simulink library "gavrt_library"  (Simulink 6.2)
libraries: xbsIndex_r3 x217, xps_library x15, casper_library x12, gavrt_library x8
(part 1 of 3)
settings Model: LastModifiedBy=Glenn

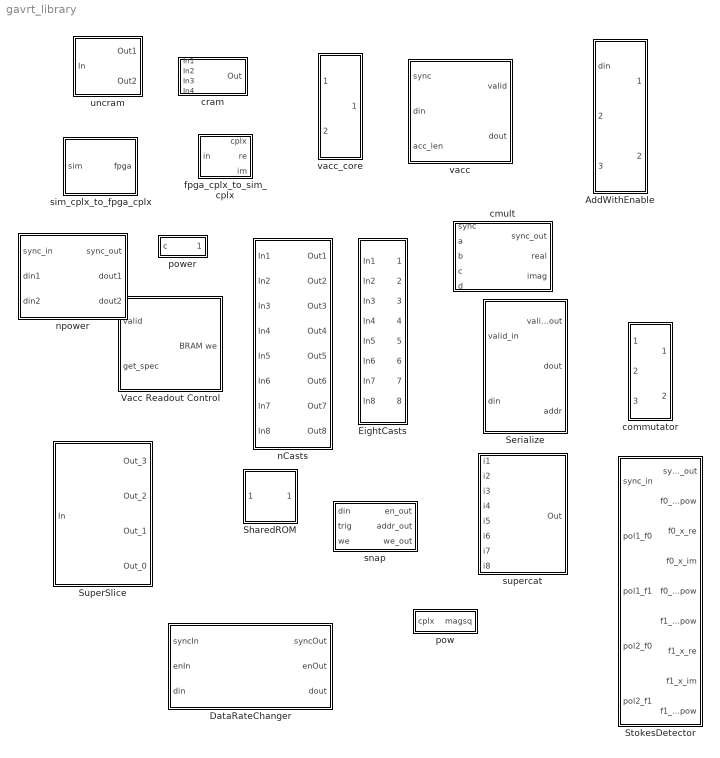
== system gavrt_library ==
  AddWithEnable : Subsystem  mask{acc_width=18, bin_pt=17, add_latency=1}
      mask prompts: acc_width "Output bit width"; bin_pt "Binary Point"; add_latency "Add Latency"
      mask help:
      | Adder with enable.
      | Used by the Addressable accumulator addracc.
      | toram = din + accen * fromram  (with latency add_latency)
      | rdout is for debugging
  DataRateChanger : Subsystem  mask(dataratechanger){input_length=3, ninputs=1, out_rate=1, in_bit_width=8, in_bin_pt=0, arith_type=0}
      mask prompts: input_length "Input Length (2^?)"; ninputs "Number of Simultaneous Inputs (2^?)"; out_rate "Output Rate (2^-?)"; in_bit_width "Input Bit Width"; in_bin_pt "Input Binary Point"; arith_type "Arithmetic Type (0=Unsigned, 1=Signed)"
      mask help:
      | Stores input data into a FIFO and then outputs the data at the specified data rate, cycling through inputs.
      | Thus if the input data looks like:
      | x0 x1 x2 x3 ...
      | y0 y1 y2 y3 ...
      | And the output rate is 2^-1, the output will look like this:
      | x0 x0 y0 y0 x1 x1 y1 y1 x2 x2 y2 y2...
      | enIn (enable In) should be high for 2^Input length clocks while the input data is valid.
      | *Currently enIn must be high in one burst of 2^Input length*
      | din should be all simultaneous inputs "crammed" together
      | enOut will be high for 2^(Input Length + Output Rate + Number of Simultaneous Inputs)
      | Arithmetic type and binary precision is only used for "uncramming" the input data
      mask init:
      | dataratechanger_init(gcb, 'input_length', input_length,...
      |     'ninputs', ninputs, ...
      |     'out_rate', out_rate,...
      |     'in_bit_width', in_bit_width,...
      |     'in_bin_pt', in_bin_pt,...
      |     'arith_type',arith_type);
  EightCasts : Subsystem  mask{nbits=0, bin_pt=0}
      mask prompts: nbits "Number of bits"; bin_pt "Binary Point"
      mask help: Eight casts to quickly connect ADC to FFT
  Serialize : Subsystem  mask(serialize){ninputs=8, in_width=8, depth=32, mux_latency=2}
      mask prompts: ninputs "Number of simultaneous inputs"; in_width "Input data bit width"; mux_latency "Mux Latency"
      mask help:
      | Takes concatenated parallel inputs and presents them one by one on dout. Designed to work with the Specacc block directly. valid_in should be high for 'depth' clocks while the data is present on din. After a short delay from when valid_in returns low, valid_out will go high and the first data will be present on dout and addr will be 0. addr increments for each subsequent output data.  dout(0) is the MSB of the first din word.
      | 'depth' must be a power of two and is the length of the input vectors. The output vector will be ninputs*depth long
      | This block can be directly connected to a Shared BRAM (provided dout is <= 32 bits).
      mask init:
      | serialize_init(gcb, ...
      |     'ninputs', ninputs, ...
      |     'in_width', in_width, ...
      |     'depth', depth, ...
      |     'mux_latency', mux_latency);
  SharedROM : Subsystem  mask(sharedrom){outwidth=327, depth=8192}
      mask prompts: outwidth "Output Bit Width"
      mask init:
      | sharedrom_init(gcb,...
      |     'outwidth', outwidth,...
      |     'depth', depth);
  StokesDetector : Subsystem  mask(stokes){bit_width=18, add_latency=2, mult_latency=3}
      mask prompts: bit_width "Bit Width"; add_latency "Add Latency"; mult_latency "Mult Latency"
      mask help: Compute cross products necessary for full stokes parameters
  SuperSlice : Subsystem  mask(superslice){slices=-1*ones(1,4)}
      mask prompts: slices "Slice pattern"
      mask help:
      | Slices the input word into consecutive outputs of arbitrary width.
      | Slice pattern should be a vector with each entry representing the width of that particular slice. The first entry is the MSB slice and the last is the LSB slice.
      | If a slice is given width -1, that slice will have a boolean output.
      | Ex: -1*ones(1,32)  -- Slice a 32 bit word into seperate boolean flags
      | [16, 8, -1*ones(1,8)] -- Slice a 32 bit word into the MSW, a byte, and the least significant 8 bits
      mask init:
      | superslice_init(gcb, 'slices', slices);
  Vacc Readout Control : Subsystem
      mask Description:
      | Designed for easily reading out vacc block with the PowerPC. Connect valid to the valid out of the vacc or serializer. Connect BRAM we to the we port of the Shared BRAM and make this bit available in a software register. Connect get_spec to a bit from a software register.
      | To read out an accumulation,
      | set get_spec high
      | wait for BRAM we to go low
      | read valid accumulation from Shared BRAM
      | set get_spec low
  cmult : Subsystem  mask(cmult_em){mult_latency=4, add_latency=3}
      mask prompts: mult_latency "Mult Latency"; add_latency "Add Latency"
      mask help: Perform a complex multiplication (a+bi)(c-di)=(ac-bd)+(ad+bc)i. Implements the logic in embedded multipliers.
  commutator : Subsystem  mask(commutator){ninputs=8, in_width=32, mux_latency=2}
      mask prompts: ninputs "Number of inputs"; in_width "Input width"; mux_latency "Mux Latency"
      mask help:
      | Used by the Serialize block.
      | din is concatenated parallel inputs. dout commutates through din from MSB to LSB.
      mask init:
      | commutator_init(gcb, ...
      |     'ninputs', ninputs, ...
      |     'in_width', in_width, ...
      |     'mux_latency', mux_latency);
  cram : Subsystem  mask(cram){num_slice=4}
      mask prompts: num_slice "Number of slices"
      mask help: Concatenates inputs together after forcing binary point to zero.
      mask init:
      | cram_init(gcb, ...
      |     'num_slice', num_slice);
  fpga_cplx_to_sim_cplx : Subsystem  mask{width=18}
      mask prompts: width "Data Width"
      mask help: Converts a Casper complex to a Simulink complex
      mask init:
      | set_param(gcb, 'AttributesFormatString', sprintf('%d_%d bit',width,width-1));
      settings: AttributesFormatString=18_17 bit
  nCasts : Subsystem  mask(ncasts){ncasts=8, arith_type=0, nbits=8, bin_pt=3}
      mask prompts: ncasts "Number of Casts"; arith_type "Arithmetic Type (0=Unsigned, 1=Signed, 2=Boolean)"; nbits "Output Bit Width"; bin_pt "Binary Point"
      mask init:
      | ncasts_init(gcb, ...
      |     'ncasts', ncasts, ...
      |     'arith_type', arith_type, ...
      |     'nbits', nbits, ...
      |     'bin_pt', bin_pt);
  npower : Subsystem  mask(npower){n_inputs=2, in_width=18, add_latency=2, mult_latency=3}
      mask prompts: n_inputs "Number of inputs"; in_width "Input Bit Width"; add_latency "Add Latency"; mult_latency "Mult Latency"
      mask init:
      | npower_init(gcb, ...
      |     'n_inputs', n_inputs, ...
      |     'in_width', in_width, ...
      |     'add_latency', add_latency, ...
      |     'mult_latency', mult_latency)
      settings: AttributesFormatString=latency=5
  pow : Subsystem  mask{bit_width=18, add_latency=2, mult_latency=3}
      mask prompts: bit_width "Bit Width"; add_latency "Add Latency"; mult_latency "Mult Latency"
  power : Subsystem  mask{BitWidth=18, add_latency=2, mult_latency=3}
      mask prompts: BitWidth "Bit Width"; add_latency "Add Latency"; mult_latency "Mult Latency"
  sim_cplx_to_fpga_cplx : Subsystem  mask{width=18}
      mask prompts: width "Data Width"
      mask help:
      | Converts a Simulink complex to fixed point and concatenates it to a Casper complex.
      | Output is two Fix_width_(width-1) numbers concatenated.
      mask init:
      | set_param(gcb, 'AttributesFormatString', sprintf('%d_%d bit',width,width-1));
      settings: AttributesFormatString=18_17 bit
  snap : Subsystem  mask(snap64){nsamples=13, latency=4}
      mask prompts: nsamples "No. of samples(2^?)"; latency "Register Latency"
      mask help:
      | The <i>snap</i> block provides a packaged solution to capturing data from
      | the FPGA fabric and making it accessible from the CPU.  The block comes in
      | 2 flavors: <i>snap</i> (which captures to a 32 bit wide Shared BRAM), and
      | <i>snap64</i> (which captures to 2x32 bit wide Shared BRAMs to effect a
      | 64 bit capture).
      | en_out provides access to the ctrl[en] bit
      | addr_out and we_out can be used to control additional BRAMs to allow for wider captures than 64 bits.
      | Register latency specifies how many levels of registers to use between the control logic and the software registers and Shared BRAMs. Adding latency can help timing when compiling at 250 MHz
      mask Help: eval('xlWeb([getenv(''MLIB_ROOT''), ''\casper_library\doc\snap_usage.html''])')
  supercat : Subsystem  mask(supercat){n=8}
      mask prompts: n "Number of Inputs"
      mask init:
      | supercat_init(gcb, 'n', n);
  uncram : Subsystem  mask(uncram){num_slice=2, slice_width=18, bin_pt=17, arith_type=1}
      mask prompts: num_slice "Number of slices"; slice_width "Slice Width"; bin_pt "Output Binary Point"; arith_type "Output Arithmetic Type (0=Unsigned, 1=Signed)"
      mask help: Takes a concatenated input and slices it up into even pieces and reinterprets them as signed fixed point numbers with a given binary point.
      mask init:
      | uncram_init(gcb, ...
      |     'num_slice', num_slice, ...
      |     'slice_width', slice_width, ...
      |     'bin_pt', bin_pt, ...
      |     'arith_type', arith_type);
      settings: AttributesFormatString=Fix_18_17
  vacc : Subsystem  mask(vacc){veclen=8, ninputs=4, max_accum=16, arith_type=0, in_bit_width=32, in_bin_pt=31, out_bit_width=48, out_bin_pt=31, register_din=0, add_latency=2, bram_latency=2, mux_latency=1}
      mask prompts: veclen "Vector Length (2^?)"; ninputs "Number of Simultaneous Vectors"; max_accum "Maximum # Accumulations (2^?)"; arith_type "Arithmetic Type (0=Unsigned, 1=Signed)"; in_bit_width "Input Bit Width"; in_bin_pt "Input Binary Point"; out_bit_width "Output Bit Width"; out_bin_pt "Output Binary Point"; register_din "Register Input Data  (1 = Enable Register Retiming on input delay)"; add_latency "Add Latency"; bram_latency "BRAM Latency"; mux_latency "Mux Latency"
      mask help:
      | Sync is expected the clock before the first data to be accumulated.
      | Use the Cram block to feed din for multiple simultaneous inputs.
      | acc_len is the number of vectors to sum.
      | valid is high while a valid accumulation is being clocked out on dout.
      | If only one sync pulse is provided, valid accumulations will repeatedly appear on dout as they become available.
      | Undesired behavior may occur if acc_len is changed without a new sync pulse.
      | Note: The output is an unsigned concatenation of the output streams. Thus, even with only one stream, the output must be recast before using.
      | Register Input Data controls the "Enable Register Retiming" parameter of the delays on 'din'.
      mask init:
      | vacc_init(gcb, ...
      |     'veclen', veclen, ...
      |     'ninputs', ninputs, ...
      |     'max_accum', max_accum, ...
      |     'arith_type', arith_type, ...
      |     'in_bit_width', in_bit_width, ...
      |     'in_bin_pt', in_bin_pt, ...
      |     'out_bit_width', out_bit_width, ...
      |     'out_bin_pt', out_bin_pt, ...
      |     'register_din', register_din, ...
      |     'add_latency', add_latency, ...
      |     'bram_latency', bram_latency, ...
      |     'mux_latency', mux_latency);
      settings: AttributesFormatString=|
      | vector length=256, inputs=4
      | max accumulations=2^16
  vacc_core : Subsystem  mask(vacc_core){veclen=16, arith_type=0, out_bit_width=14, out_bin_pt=0, add_latency=2, bram_latency=2, mux_latency=1}
      mask prompts: veclen "Vector Length"; arith_type "Arithmetic Type (0=Unsigned, 1=Signed)"; out_bit_width "Output Bit Width"; out_bin_pt "Output Binary Point"; add_latency "Add Latency"; bram_latency "BRAM Latency"; mux_latency "Mux Latency"
      mask help:
      | Currently only Signed arithmetic supported
      | acc_en = 0 --> Load a vector (start a new accumulation)
      | acc_en = 1 --> Accumulate
      mask init:
      | vacc_core_init(gcb, ...
      |     'veclen', veclen, ...
      |     'arith_type', arith_type, ...
      |     'out_bit_width', out_bit_width, ...
      |     'out_bin_pt', out_bin_pt, ...
      |     'add_latency', add_latency, ...
      |     'bram_latency', bram_latency, ...
      |     'mux_latency', mux_latency);

== system gavrt_library/AddWithEnable ==
  din : Inport  Port=1  LatchInput=off
  accen : Inport  Port=2  LatchInput=off
  fromram : Inport  Port=3  LatchInput=off
  AddSub : xbsIndex_r3/AddSub  mode=Addition  precision=Full  arith_type=Unsigned  n_bits=8  bin_pt=2  quantization=Truncate  overflow=Wrap  latency=add_latency  explicit_period=off  period=1  use_carryin=off  use_carryout=off  en=off  dbl_ovrd=off  show_param=on  use_core=on  pipeline=on  use_rpm=on  gen_core=off
      settings: xl_area=[0, 0, 0, 0, 0, 0, 0]
  Constant1 : xbsIndex_r3/Constant  const=0  equ=P=C  arith_type="Signed  (2's comp)"  n_bits=acc_width  bin_pt=bin_pt  opselect=C  inp2=PCIN>>17  opr=+  inp1=P  carry=CIN  iostate=0  explicit_period=on  period=1  dbl_ovrd=off
  Convert2 : xbsIndex_r3/Convert  arith_type="Signed  (2's comp)"  n_bits=acc_width  bin_pt=bin_pt  quantization=Truncate  overflow=Wrap  latency=0  explicit_period=off  period=1  dbl_ovrd=off  show_param=off  inserted_by_tool=off  pipeline=off
      settings: xl_area=[0, 0, 0, 0, 0, 0, 0]
  Mux : xbsIndex_r3/Mux  inputs=2  precision=Full  arith_type="Signed  (2's comp)"  n_bits=8  bin_pt=2  quantization=Truncate  overflow=Wrap  latency=0  explicit_period=off  period=1  en=off  dbl_ovrd=off  show_param=off  mux_type=off  use_rpm=off  gen_core=off
      settings: xl_area=[0, 0, 0, 0, 0, 0, 0]
  Reinterpret : xbsIndex_r3/Reinterpret  force_arith_type=on  arith_type="Signed  (2's comp)"  force_bin_pt=on  bin_pt=bin_pt  force_valid=on
  Reinterpret1 : xbsIndex_r3/Reinterpret  force_arith_type=on  arith_type=Unsigned  force_bin_pt=on  bin_pt=0  force_valid=on
  toram : Outport
  rdout : Outport  Port=2
  wires:
  Constant1/1 -> Mux/2
  Reinterpret/1 -> Mux/3, rdout/1
  Mux/1 -> AddSub/2
  AddSub/1 -> Convert2/1
  Convert2/1 -> Reinterpret1/1
  din/1 -> AddSub/1
  accen/1 -> Mux/1
  Reinterpret1/1 -> toram/1
  fromram/1 -> Reinterpret/1

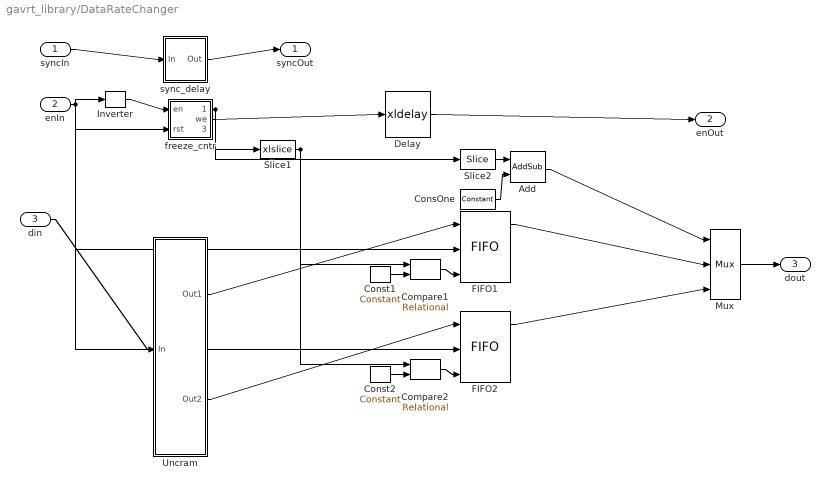
== system gavrt_library/DataRateChanger ==
  syncIn : Inport  Port=1  LatchInput=off
  enIn : Inport  Port=2  LatchInput=off
  din : Inport  Port=3  LatchInput=off
  Add : xbsIndex_r3/AddSub  mode=Addition  precision=User Defined  arith_type=Unsigned  n_bits=1  bin_pt=0  quantization=Truncate  overflow=Wrap  latency=0  explicit_period=off  period=1  use_carryin=off  use_carryout=off  en=off  dbl_ovrd=off  show_param=off  use_core=on  pipeline=off  use_rpm=on  gen_core=off
      settings: xl_area=[0, 0, 0, 0, 0, 0, 0]
  Compare1 : xbsIndex_r3/Relational  mode=a=b  latency=0  explicit_period=off  period=1  en=off  dbl_ovrd=off  show_param=off
      settings: xl_area=[0, 0, 0, 0, 0, 0, 0]
  Compare2 : xbsIndex_r3/Relational  mode=a=b  latency=0  explicit_period=off  period=1  en=off  dbl_ovrd=off  show_param=off
      settings: xl_area=[0, 0, 0, 0, 0, 0, 0]
  ConsOne : xbsIndex_r3/Constant  const=1  equ=P=C  arith_type=Unsigned  n_bits=1  bin_pt=0  opselect=C  inp2=PCIN>>17  opr=+  inp1=P  carry=CIN  iostate=0  explicit_period=off  period=1  dbl_ovrd=off
  Const1 : xbsIndex_r3/Constant  const=1  equ=P=C  arith_type=Unsigned  n_bits=2  bin_pt=0  opselect=C  inp2=PCIN>>17  opr=+  inp1=P  carry=CIN  iostate=0  explicit_period=off  period=1  dbl_ovrd=off
  Const2 : xbsIndex_r3/Constant  const=3  equ=P=C  arith_type=Unsigned  n_bits=2  bin_pt=0  opselect=C  inp2=PCIN>>17  opr=+  inp1=P  carry=CIN  iostate=0  explicit_period=off  period=1  dbl_ovrd=off
  Delay : S-Function  AncestorBlock=xbsIndex_r3/Delay  FunctionName=xldelay  Parameters=sfcn_mwsv__  mask(Xilinx Delay Block){latency=3, reg_retiming=off, explicit_period=off, period=1, en=off, accept_only_valid=off, init_zero=on, dbl_ovrd=off, show_param=off, xl_area=[0, 0, 0, 0, 0, 0, 0], xl_use_area=off}
      mask prompts: reg_retiming "Enable Register Retiming"; explicit_period "Use Explicit Sample Period"; period "Sample Period  (use -1 to inherit first known input period)"; en "Provide Enable Port"; accept_only_valid "Shift In Only Valid Data"; init_zero "Initialize with Zeros (otherwise Invalid)"; dbl_ovrd "Override with Doubles"; show_param "---------------------- Show Implementation Parameters -----------------------------------------------------------------------------------"; xl_area "FPGA Area [Slices, FFs, BRAMs, LUTs, IOBs, Emb. Mults, TBUFs]"; xl_use_area "Use Area Above For Estimation"
      mask help:
      | Delay line having  configurable length.
      |
      | Hardware notes: A delay line is a chain, each link of which is an SRL16 followed by a flip-flop. If register retiming is enabled, the delay line is a chain of flip-flops.
      mask init:
      | rst = 0;
      | [enPortNum,enPortStr,rstPortNum,rstPortStr] = xlport_en_rst(en,rst,2);
      | str = sprintf('-%d',latency);
      | [designRoot, family, part, speed, package, simulinkPeriod, sysclkPeriod, dbl_ovrd, trimVbit] = xlSysgenSettings(gcb,1,1);
      | [bg,fg] = xlcmap('XBlock',dbl_ovrd);
      | iPos = get_param(gcb,'Position');
      | iWidth=iPos(3)-iPos(1); iHeight=iPos(4)-iPos(2);
      | iCx=iWidth/2;
      | iCy=iHeight/2;
      | [logoX, logoY] = xlogo(iPos);
      | 
      | 
      | % one time added for param list
      | dblOvrd = dbl_ovrd;
      | vOnly = accept_only_valid;
      | initZero = init_zero;
      | precision0 = 1;
      | z0 = [0 0 1 1 1];
      | explicitClk = explicit_period;
      | 
      | hasRST = rst;
      | hasEN = en;
      | % just pass everything to s-function
      | sfcn_mwsv__ = get_param(gcb, 'MaskWSVariables');
      mask Help: eval('xlWeb(xlhtmldoclink(''Delay''))');
      mask CallbackString: ||xlMagicCallback||||||xlShowIPCallback||
      mask Display:
      | patch([0 iWidth iWidth 0],[0 0 iHeight iHeight] , bg);
      | patch(logoX,logoY , fg);
      | text(iCx-6,iCy,'z');
      | text(iCx,iCy+4,str);
      | port_label('input',enPortNum,enPortStr);
      | ;plot([0 0 iWidth iWidth 0], [0 iHeight iHeight 0 0]);
  FIFO1 : xbsIndex_r3/FIFO  depth=16  percent_nbits=1  store_only_valid=on  init_zero=on  explicit_period=off  period=1  rst=off  en=off  use_almost_empty=off  almost_empty_offset=6  use_almost_full=off  almost_full_offset=6  dbl_ovrd=off  show_param=off  mem_type=Block RAM  gen_core=off
      settings: xl_area=[0, 0, 0, 0, 0, 0, 0]
  FIFO2 : xbsIndex_r3/FIFO  depth=16  percent_nbits=1  store_only_valid=on  init_zero=on  explicit_period=off  period=1  rst=off  en=off  use_almost_empty=off  almost_empty_offset=6  use_almost_full=off  almost_full_offset=6  dbl_ovrd=off  show_param=off  mem_type=Block RAM  gen_core=off
      settings: xl_area=[0, 0, 0, 0, 0, 0, 0]
  Inverter : xbsIndex_r3/Inverter  latency=0  explicit_period=off  period=1  en=off  dbl_ovrd=off  show_param=off
      settings: xl_area=[0, 0, 0, 0, 0, 0, 0]
  Mux : xbsIndex_r3/Mux  inputs=2  precision=Full  arith_type="Signed  (2's comp)"  n_bits=8  bin_pt=2  quantization=Truncate  overflow=Wrap  latency=1  explicit_period=off  period=1  en=off  dbl_ovrd=off  show_param=off  mux_type=off  use_rpm=off  gen_core=off
      settings: xl_area=[0, 0, 0, 0, 0, 0, 0]
  Slice1 : S-Function  AncestorBlock=xbsIndex_r3/Slice  FunctionName=xlslice  Parameters=sfcn_mwsv__  mask(Xilinx Slice Block){mode=Lower Bit Location + Width, nbits=2, bit1=-3, base1=MSB of Input, bit0=0, base0=LSB of Input, boolean_output=off, explicit_period=off, period=1, dbl_ovrd=off}
      mask prompts: mode "Specify Range As"; nbits "Width of Slice (number of bits)"; bit1 "Offset of Top Bit"; base1 "Relative To"; bit0 "Offset of Bottom Bit"; base0 "Relative To"; boolean_output "Boolean Output"; explicit_period "Use Explicit Sample Period"; period "Sample Period"; dbl_ovrd "Override with Doubles"
      mask help:
      | Bit slice extractor.  Extracts a given range of bits from each input sample and presents it at the output.  The output type is ordinarily unsigned with binary point at zero, but can be Boolean when the slice is one bit wide.
      |
      | Hardware notes: In hardware this block costs nothing.
      mask init:
      | [designRoot, family, part, speed, package, simulinkPeriod, sysclkPeriod, dbl_ovrd, trimVbit] = xlSysgenSettings(gcb,1,1);
      | dbl_ovrdStr = '';
      | [bg,fg]=xlcmap('XBlock',dbl_ovrd);
      | iPos = get_param(gcb,'Position');
      | iWidth=iPos(3)-iPos(1); iHeight=iPos(4)-iPos(2);
      | iCx=iWidth/2;
      | iCy=iHeight/2;
      | [logoX, logoY] = xlogo(iPos);
      | 
      | 
      | % one time added for param list
      | bo = boolean_output;
      | dblOvrd = dbl_ovrd;
      | precision0 = 1;
      | z0 = [nbits 0 1 1 1];
      | explicitClk = explicit_period;
      | 
      | 
      | % just pass everything to s-function
      | sfcn_mwsv__ = get_param(gcb, 'MaskWSVariables');
      mask Help: eval('xlWeb(xlhtmldoclink(''Slice''))');
      mask StyleString: popup(Two Bit Locations|Upper Bit Location + Width|Lower Bit Location + Width),edit,edit,popup(LSB of Input|Binary Point of Input|MSB of Input),edit,popup(LSB of Input|Binary Point of Input|MSB of Input),checkbox,checkbox,edit,checkbox
      mask CallbackString: xlslice_callback|||||||xlMagicCallback||
      mask Display:
      | patch([0 iWidth iWidth 0],[0 0 iHeight iHeight] , bg);
      | patch(logoX,logoY , fg);
      | port_label('output',1,'[a:b]');
      | 
      | ;plot([0 0 iWidth iWidth 0], [0 iHeight iHeight 0 0]);
  Slice2 : xbsIndex_r3/Slice  mode=Lower Bit Location + Width  nbits=1  bit1=0  base1=MSB of Input  bit0=1  base0=LSB of Input  boolean_output=off  explicit_period=off  period=1  dbl_ovrd=off
  Uncram : Subsystem  AncestorBlock=gavrt_library/uncram  mask(uncram){num_slice=2, slice_width=8, bin_pt=0, arith_type=0}
      mask prompts: num_slice "Number of slices"; slice_width "Slice Width"; bin_pt "Output Binary Point"; arith_type "Output Arithmetic Type (0=Unsigned, 1=Signed)"
      mask help: Takes a concatenated input and slices it up into even pieces and reinterprets them as signed fixed point numbers with a given binary point.
      mask init:
      | uncram_init(gcb, ...
      |     'num_slice', num_slice, ...
      |     'slice_width', slice_width, ...
      |     'bin_pt', bin_pt, ...
      |     'arith_type', arith_type);
      settings: AttributesFormatString=UFix_8_0
  freeze_cntr : Subsystem  AncestorBlock=casper_library/Misc/freeze_cntr  mask(freeze_cntr){CounterBits=5}
      mask prompts: CounterBits "Counter Length (2^?)"
      mask help:
      | A freeze counter is an enabled counter which holds its final value (regardless of enables)
      | until it is reset.
      mask Help: eval('xlWeb([getenv(''MLIB_ROOT''), ''\casper_library\doc\freeze_cntr_usage.html''])')
  sync_delay : Subsystem  AncestorBlock=casper_library/Delays/sync_delay  mask(sync_delay){DelayLen=11}
      mask prompts: DelayLen "Delay Length:"
      mask help: Delay an infrequent boolean pulse by the specified number of clocks.
      mask init:
      | BitWidth = max(2, ceil(log2(DelayLen+1)));
      | UseCounter = 1;
      | if DelayLen == 0,
      | 	UseCounter = 0;
      | end
      mask Help: eval('xlWeb([getenv(''MLIB_ROOT''), ''\casper_library\doc\sync_delay_usage.html''])')
      mask Display: fprintf('Z^-%d', DelayLen)
  syncOut : Outport
  enOut : Outport  Port=2
  dout : Outport  Port=3
  wires:
  FIFO2/1 -> Mux/3
  Uncram/2(Out2) -> FIFO2/1
  Compare2/1 -> FIFO2/3
  Const2/1 -> Compare2/2
  Slice1/1 -> Compare2/1, Compare1/1
  FIFO1/1 -> Mux/2
  Uncram/1(Out1) -> FIFO1/1
  Compare1/1 -> FIFO1/3
  Const1/1 -> Compare1/2
  Add/1 -> Mux/1
  ConsOne/1 -> Add/2
  Slice2/1 -> Add/1
  Mux/1 -> dout/1
  din/1 -> Uncram/1(In)
  freeze_cntr/1(addr) -> Slice2/1, Slice1/1
  Delay/1 -> enOut/1
  freeze_cntr/2(we) -> Delay/1
  Inverter/1 -> freeze_cntr/1(en)
  enIn/1 -> FIFO2/2, FIFO1/2, freeze_cntr/2(rst), Inverter/1
  sync_delay/1(Out) -> syncOut/1
  syncIn/1 -> sync_delay/1(In)

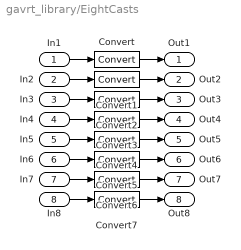
== system gavrt_library/EightCasts ==
  In1 : Inport  Port=1  LatchInput=off
  In2 : Inport  Port=2  LatchInput=off
  In3 : Inport  Port=3  LatchInput=off
  In4 : Inport  Port=4  LatchInput=off
  In5 : Inport  Port=5  LatchInput=off
  In6 : Inport  Port=6  LatchInput=off
  In7 : Inport  Port=7  LatchInput=off
  In8 : Inport  Port=8  LatchInput=off
  Convert{,1..7} (8 alike) : xbsIndex_r3/Convert  arith_type="Signed  (2's comp)"  n_bits=nbits  bin_pt=bin_pt  quantization=Truncate  overflow=Wrap  latency=0  explicit_period=off  period=1  dbl_ovrd=off  show_param=off  inserted_by_tool=off  pipeline=off
      settings: xl_area=[0, 0, 0, 0, 0, 0, 0]
  Out1 : Outport
  Out2 : Outport  Port=2
  Out3 : Outport  Port=3
  Out4 : Outport  Port=4
  Out5 : Outport  Port=5
  Out6 : Outport  Port=6
  Out7 : Outport  Port=7
  Out8 : Outport  Port=8
  wires:
  Convert7/1 -> Out8/1
  In8/1 -> Convert7/1
  Convert6/1 -> Out7/1
  In7/1 -> Convert6/1
  Convert5/1 -> Out6/1
  In6/1 -> Convert5/1
  Convert4/1 -> Out5/1
  In5/1 -> Convert4/1
  Convert3/1 -> Out4/1
  In4/1 -> Convert3/1
  Convert2/1 -> Out3/1
  In3/1 -> Convert2/1
  Convert1/1 -> Out2/1
  In2/1 -> Convert1/1
  Convert/1 -> Out1/1
  In1/1 -> Convert/1

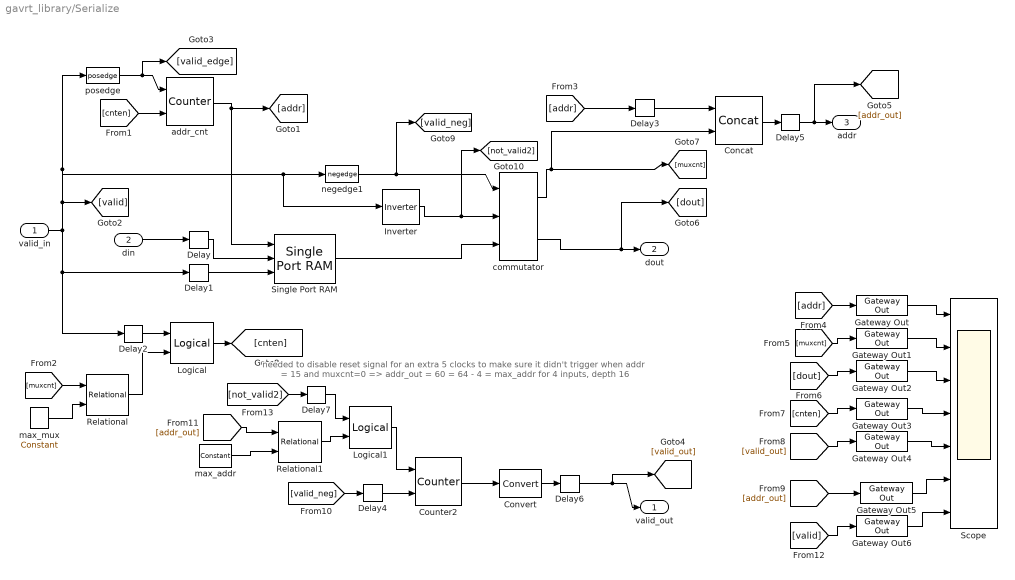
== system gavrt_library/Serialize ==
  note: needed to disable reset signal for
      | an extra 5 clocks to make sure it didn't
      | trigger when addr = 15 and muxcnt=0 =>
      | addr_out = 60 = 64 - 4 = max_addr for
      | 4 inputs, depth 16
  valid_in : Inport  Port=1  LatchInput=off
  din : Inport  Port=2  LatchInput=off
  Concat : xbsIndex_r3/Concat  num_inputs=2  explicit_period=off  period=1  dbl_ovrd=off
  Convert : xbsIndex_r3/Convert  arith_type=Boolean  n_bits=8  bin_pt=6  quantization=Truncate  overflow=Wrap  latency=0  explicit_period=off  period=1  dbl_ovrd=off  show_param=off  inserted_by_tool=off  pipeline=off
      settings: xl_area=[0, 0, 0, 0, 0, 0, 0]
  Counter2 : xbsIndex_r3/Counter  cnt_type=Free Running  n_bits=1  bin_pt=0  arith_type=Unsigned  start_count=0  cnt_to=Inf  cnt_by_val=1  operation=Up  explicit_period=off  period=1  load_pin=off  rst=on  en=on  dbl_ovrd=off  show_param=off  use_rpm=on  gen_core=off
      settings: xl_area=[0, 0, 0, 0, 0, 0, 0]
  Delay{,1..4} (5 alike) : xbsIndex_r3/Delay  latency=1  reg_retiming=off  explicit_period=off  period=1  en=off  accept_only_valid=off  init_zero=on  dbl_ovrd=off  show_param=off
      settings: xl_area=[0, 0, 0, 0, 0, 0, 0]
  Delay5 : xbsIndex_r3/Delay  latency=2  reg_retiming=on  explicit_period=off  period=1  en=off  accept_only_valid=off  init_zero=on  dbl_ovrd=off  show_param=off
      settings: xl_area=[0, 0, 0, 0, 0, 0, 0]
  Delay6 : xbsIndex_r3/Delay  latency=2  reg_retiming=on  explicit_period=off  period=1  en=off  accept_only_valid=off  init_zero=on  dbl_ovrd=off  show_param=off
      settings: xl_area=[0, 0, 0, 0, 0, 0, 0]
  Delay7 : xbsIndex_r3/Delay  latency=3  reg_retiming=off  explicit_period=off  period=1  en=off  accept_only_valid=off  init_zero=on  dbl_ovrd=off  show_param=off
      settings: xl_area=[0, 0, 0, 0, 0, 0, 0]
  Gateway Out{,1..6} (7 alike) : xbsIndex_r3/Gateway Out  output_type=Double  nbits=8  bin_pt=6  arith_type=Boolean  quantization=Truncate  overflow=Wrap  hdl_port=off  timing_constraint=None  locs_specified=off  LOCs={}  needs_fixed_name=off  show_param=off
      settings: xl_area=[0, 0, 0, 0, 0, 0, 0]
  Inverter : xbsIndex_r3/Inverter  latency=2  explicit_period=off  period=1  en=off  dbl_ovrd=off  show_param=off
      settings: xl_area=[0, 0, 0, 0, 0, 0, 0]
  Logical : xbsIndex_r3/Logical  logical_function=OR  inputs=2  precision=Full  arith_type=Unsigned  n_bits=8  bin_pt=2  align_bp=on  latency=0  explicit_period=off  period=1  en=off  dbl_ovrd=off  show_param=off
      settings: xl_area=[0, 0, 0, 0, 0, 0, 0]
  Logical1 : xbsIndex_r3/Logical  logical_function=AND  inputs=2  precision=Full  arith_type=Unsigned  n_bits=8  bin_pt=2  align_bp=on  latency=0  explicit_period=off  period=1  en=off  dbl_ovrd=off  show_param=off
      settings: xl_area=[0, 0, 0, 0, 0, 0, 0]
  Relational : xbsIndex_r3/Relational  mode=a=b  latency=1  explicit_period=off  period=1  en=off  dbl_ovrd=off  show_param=off
      settings: xl_area=[0, 0, 0, 0, 0, 0, 0]
  Relational1 : xbsIndex_r3/Relational  mode=a=b  latency=1  explicit_period=off  period=1  en=off  dbl_ovrd=off  show_param=off
      settings: xl_area=[0, 0, 0, 0, 0, 0, 0]
  Scope : Scope  NumInputPorts=7
      settings: TimeRange=256  YMin=-5~-5~-5~-5~-5~-5~-5  YMax=5~5~5~5~5~5~5
  Single Port RAM : xbsIndex_r3/Single Port RAM  depth=32  initVector=sin(pi*(0:15)/16)  write_mode=Read After Write  latency=1  init_zero=on  explicit_period=off  period=1  rst=off  init_reg=0  en=off  dbl_ovrd=off  show_param=off  distributed_mem=off  use_rpm=off  gen_core=off
      settings: xl_area=[0, 0, 0, 0, 0, 0, 0]
  addr_cnt : xbsIndex_r3/Counter  cnt_type=Free Running  n_bits=5  bin_pt=0  arith_type=Unsigned  start_count=0  cnt_to=Inf  cnt_by_val=1  operation=Up  explicit_period=off  period=1  load_pin=off  rst=on  en=on  dbl_ovrd=off  show_param=off  use_rpm=on  gen_core=off
      settings: xl_area=[0, 0, 0, 0, 0, 0, 0]
  commutator : gavrt_library/commutator  ninputs=8  in_width=8  mux_latency=2
  max_addr : xbsIndex_r3/Constant  const=252  equ=P=C  arith_type=Unsigned  n_bits=8  bin_pt=0  opselect=C  inp2=PCIN>>17  opr=+  inp1=P  carry=CIN  iostate=0  explicit_period=on  period=1  dbl_ovrd=off
  max_mux : xbsIndex_r3/Constant  const=5  equ=P=C  arith_type=Unsigned  n_bits=3  bin_pt=0  opselect=C  inp2=PCIN>>17  opr=+  inp1=P  carry=CIN  iostate=0  explicit_period=on  period=1  dbl_ovrd=off
  negedge1 : casper_library/Misc/negedge  Tag=Rising Edge Detector
  posedge : casper_library/Misc/posedge  Tag=Rising Edge Detector
  valid_out : Outport
  dout : Outport  Port=2
  addr : Outport  Port=3
  wires:
  [not_valid2] -> Delay7/1
  Delay7/1 -> Logical1/1
  Relational1/1 -> Logical1/2
  Logical1/1 -> Counter2/1
  Gateway Out6/1 -> Scope/7
  [valid] -> Gateway Out6/1
  valid_in/1 -> [valid], negedge1/1, Inverter/1, posedge/1, Delay1/1, Delay2/1
  posedge/1 -> addr_cnt/1, [valid_edge]
  addr_cnt/1 -> Single Port RAM/1, [addr]
  din/1 -> Delay/1
  Delay/1 -> Single Port RAM/2
  Delay1/1 -> Single Port RAM/3
  Single Port RAM/1 -> commutator/3
  commutator/2 -> dout/1, [dout]
  negedge1/1 -> [valid_neg], commutator/1
  Inverter/1 -> [not_valid2], commutator/2
  [addr] -> Delay3/1
  Concat/1 -> Delay5/1
  Gateway Out/1 -> Scope/1
  Gateway Out1/1 -> Scope/2
  Gateway Out2/1 -> Scope/3
  Gateway Out3/1 -> Scope/4
  Gateway Out4/1 -> Scope/5
  [addr] -> Gateway Out/1
  [muxcnt] -> Gateway Out1/1
  [dout] -> Gateway Out2/1
  [cnten] -> Gateway Out3/1
  [valid_out] -> Gateway Out4/1
  Delay2/1 -> Logical/1
  Logical/1 -> [cnten]
  [cnten] -> addr_cnt/2
  [muxcnt] -> Relational/1
  max_mux/1 -> Relational/2
  Relational/1 -> Logical/2
  [addr_out] -> Gateway Out5/1
  Gateway Out5/1 -> Scope/6
  Delay3/1 -> Concat/1
  [valid_neg] -> Delay4/1
  Delay4/1 -> Counter2/2
  [addr_out] -> Relational1/1
  max_addr/1 -> Relational1/2
  Counter2/1 -> Convert/1
  Delay5/1 -> addr/1, [addr_out]
  Delay6/1 -> [valid_out], valid_out/1
  Convert/1 -> Delay6/1
  commutator/1 -> Concat/2, [muxcnt]

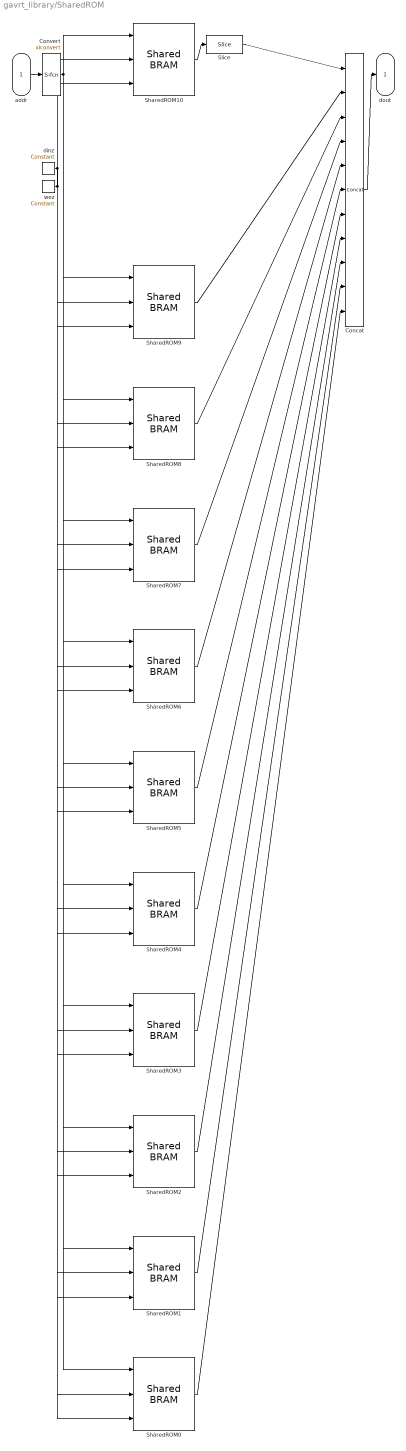
== system gavrt_library/SharedROM ==
  addr : Inport  Port=1  LatchInput=off
  Concat : xbsIndex_r3/Concat  num_inputs=11  explicit_period=off  period=1  dbl_ovrd=off
  Convert : S-Function  AncestorBlock=xbsIndex_r3/Convert  FunctionName=xlconvert  Parameters=sfcn_mwsv__  mask(Xilinx Converter Block){arith_type=Unsigned, n_bits=13, bin_pt=0, quantization=Truncate, overflow=Wrap, latency=0, explicit_period=off, period=1, dbl_ovrd=off, show_param=off, inserted_by_tool=off, pipeline=off, xl_area=[0, 0, 0, 0, 0, 0, 0], xl_use_area=off}
      mask prompts: arith_type "Output Type"; n_bits "Number of Bits"; bin_pt "Binary Point"; quantization "Quantization Behavior"; overflow "Overflow Behavior"; explicit_period "Use Explicit Sample Period"; period "Sample Period"; dbl_ovrd "Override with Doubles"; show_param "---------------------- Show Implementation Parameters -----------------------------------------------------------------------------------"; inserted_by_tool "Hidden Parameter:  inserted_by_tool"; pipeline "Pipeline to Greatest Extent Possible"; xl_area "FPGA Area [Slices, FFs, BRAMs, LUTs, IOBs, Emb. Mults, TBUFs]"; xl_use_area "Use Area Above For Estimation"
      mask help:
      | Type conversion block. The input is presented at the output after quantization and overflow effects.
      |
      | Hardware notes: Additional hardware is used when rounding or saturation is selected and output width is less than the input width.
      mask init:
      | [designRoot, family, part, speed, package, simulinkPeriod, sysclkPeriod, dbl_ovrd, trimVbit] = xlSysgenSettings(gcb,1,1);
      | if (arith_type==1)
      |   bool = 1;
      | else
      |   bool = 0;
      |   arith_type = arith_type-1;
      | end
      | zstr=''; zpstr='';
      | if latency > 0
      |   zstr = 'z';
      |   zpstr = sprintf('-%d', latency);
      | end
      | [bg,fg] = xlcmap('XBlock',dbl_ovrd);
      | if (inserted_by_tool)
      |   bg = [1.00 0.50 0.25];
      | end
      | iPos = get_param(gcb,'Position');
      | iWidth=iPos(3)-iPos(1); iHeight=iPos(4)-iPos(2);
      | iCx=iWidth/2;
      | iCy=iHeight/2;
      | [logoX, logoY] = xlogo(iPos);
      | zstrx = 0.45*iWidth-11; if (zstrx<3) zstrx=3; end
      | zstry = 0.36*iHeight-7; if (zstry<3) zstry=3; end
      | 
      | 
      | % one time added for param list
      | dblOvrd = dbl_ovrd;
      | precision0 = 2;
      | z0 = [n_bits bin_pt arith_type quantization overflow];
      | explicitClk = explicit_period;
      | 
      | 
      | % just pass everything to s-function
      | sfcn_mwsv__ = get_param(gcb, 'MaskWSVariables');
      mask Help: eval('xlWeb(xlhtmldoclink(''Convert''))');
      mask StyleString: popup(Boolean|Unsigned|Signed  (2's comp)),edit,edit,popup(Truncate|Round  (unbiased: +/- Inf)|Round  (unbiased: Even Values)),popup(Wrap|Saturate|Error),edit,checkbox,edit,checkbox,checkbox,checkbox,checkbox,edit,checkbox
      mask CallbackString: xlconvertCallback||||||xlMagicCallback|||xlShowIPCallback||||
      mask Display:
      | patch([0 iWidth iWidth 0],[0 0 iHeight iHeight] , bg);
      | patch(logoX,logoY , fg);
      | text(zstrx,zstry,zstr);
      | text(zstrx+5,zstry+5,zpstr);
      | port_label('output',1,'cast');
      | plot([0 0 iWidth iWidth 0], [0 iHeight iHeight 0 0]);
  SharedROM{0..10} (11 alike) : xps_library/Shared BRAM  Tag=xps:bram  arith_type=Unsigned  addr_width=13  data_width=32  data_bin_pt=0  init_vals=[1:2^11]  sample_rate=1
  Slice : xbsIndex_r3/Slice  mode=Lower Bit Location + Width  nbits=7  bit1=0  base1=MSB of Input  bit0=0  base0=LSB of Input  boolean_output=off  explicit_period=off  period=1  dbl_ovrd=off
  dinz : xbsIndex_r3/Constant  const=0  equ=P=C  arith_type=Unsigned  n_bits=32  bin_pt=0  opselect=C  inp2=PCIN>>17  opr=+  inp1=P  carry=CIN  iostate=0  explicit_period=off  period=1  dbl_ovrd=off
  wez : xbsIndex_r3/Constant  const=0  equ=P=C  arith_type=Boolean  n_bits=1  bin_pt=0  opselect=C  inp2=PCIN>>17  opr=+  inp1=P  carry=CIN  iostate=0  explicit_period=off  period=1  dbl_ovrd=off
  dout : Outport
  wires:
  addr/1 -> Convert/1
  Concat/1 -> dout/1
  Convert/1 -> SharedROM9/1, SharedROM8/1, SharedROM7/1, SharedROM6/1, SharedROM5/1, SharedROM4/1, SharedROM3/1, SharedROM2/1, SharedROM1/1, SharedROM0/1, SharedROM10/1
  dinz/1 -> SharedROM9/2, SharedROM8/2, SharedROM7/2, SharedROM6/2, SharedROM5/2, SharedROM4/2, SharedROM3/2, SharedROM2/2, SharedROM1/2, SharedROM0/2, SharedROM10/2
  wez/1 -> SharedROM9/3, SharedROM8/3, SharedROM7/3, SharedROM6/3, SharedROM5/3, SharedROM4/3, SharedROM3/3, SharedROM2/3, SharedROM1/3, SharedROM0/3, SharedROM10/3
  SharedROM9/1 -> Concat/2
  SharedROM8/1 -> Concat/3
  SharedROM7/1 -> Concat/4
  SharedROM6/1 -> Concat/5
  SharedROM5/1 -> Concat/6
  SharedROM4/1 -> Concat/7
  SharedROM3/1 -> Concat/8
  SharedROM2/1 -> Concat/9
  SharedROM1/1 -> Concat/10
  SharedROM0/1 -> Concat/11
  SharedROM10/1 -> Slice/1
  Slice/1 -> Concat/1

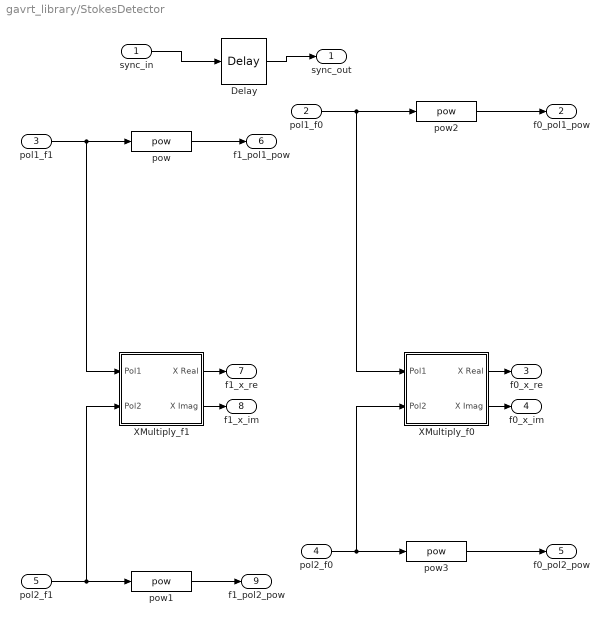
== system gavrt_library/StokesDetector ==
  sync_in : Inport  Port=1  LatchInput=off
  pol1_f0 : Inport  Port=2  LatchInput=off
  pol1_f1 : Inport  Port=3  LatchInput=off
  pol2_f0 : Inport  Port=4  LatchInput=off
  pol2_f1 : Inport  Port=5  LatchInput=off
  Delay : xbsIndex_r3/Delay  latency=add_latency + mult_latency  reg_retiming=off  explicit_period=off  period=1  en=off  accept_only_valid=off  init_zero=on  dbl_ovrd=off  show_param=off
      settings: xl_area=[0, 0, 0, 0, 0, 0, 0]
  XMultiply_f0 : Subsystem
  XMultiply_f1 : Subsystem
  pow{,1..3} (4 alike) : gavrt_library/pow  bit_width=bit_width  add_latency=add_latency  mult_latency=mult_latency
  sync_out : Outport
  f0_pol1_pow : Outport  Port=2
  f0_x_re : Outport  Port=3
  f0_x_im : Outport  Port=4
  f0_pol2_pow : Outport  Port=5
  f1_pol1_pow : Outport  Port=6
  f1_x_re : Outport  Port=7
  f1_x_im : Outport  Port=8
  f1_pol2_pow : Outport  Port=9
  wires:
  pol2_f1/1 -> XMultiply_f1/2(Pol2), pow1/1
  pol1_f0/1 -> XMultiply_f0/1(Pol1), pow2/1
  pol2_f0/1 -> XMultiply_f0/2(Pol2), pow3/1
  pol1_f1/1 -> XMultiply_f1/1(Pol1), pow/1
  pow2/1 -> f0_pol1_pow/1
  pow/1 -> f1_pol1_pow/1
  XMultiply_f0/1(X Real) -> f0_x_re/1
  XMultiply_f1/1(X Real) -> f1_x_re/1
  XMultiply_f0/2(X Imag) -> f0_x_im/1
  XMultiply_f1/2(X Imag) -> f1_x_im/1
  pow3/1 -> f0_pol2_pow/1
  pow1/1 -> f1_pol2_pow/1
  sync_in/1 -> Delay/1
  Delay/1 -> sync_out/1

== system gavrt_library/SuperSlice ==
  In : Inport  Port=1  LatchInput=off
  Slice1 : xbsIndex_r3/Slice  mode=Upper Bit Location + Width  nbits=1  bit1=-3  base1=MSB of Input  bit0=0  base0=LSB of Input  boolean_output=on  explicit_period=off  period=1  dbl_ovrd=off
  Slice2 : xbsIndex_r3/Slice  mode=Upper Bit Location + Width  nbits=1  bit1=-2  base1=MSB of Input  bit0=0  base0=LSB of Input  boolean_output=on  explicit_period=off  period=1  dbl_ovrd=off
  Slice3 : xbsIndex_r3/Slice  mode=Upper Bit Location + Width  nbits=1  bit1=-1  base1=MSB of Input  bit0=0  base0=LSB of Input  boolean_output=on  explicit_period=off  period=1  dbl_ovrd=off
  Slice4 : xbsIndex_r3/Slice  mode=Upper Bit Location + Width  nbits=1  bit1=0  base1=MSB of Input  bit0=0  base0=LSB of Input  boolean_output=on  explicit_period=off  period=1  dbl_ovrd=off
  Out_3 : Outport
  Out_2 : Outport  Port=2
  Out_1 : Outport  Port=3
  Out_0 : Outport  Port=4
  wires:
  In/1 -> Slice1/1, Slice2/1, Slice3/1, Slice4/1
  Slice1/1 -> Out_3/1
  Slice2/1 -> Out_2/1
  Slice3/1 -> Out_1/1
  Slice4/1 -> Out_0/1

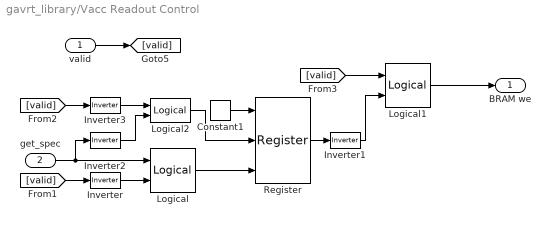
== system gavrt_library/Vacc Readout Control ==
  valid : Inport  Port=1  LatchInput=off
  get_spec : Inport  Port=2  LatchInput=off
  Constant1 : xbsIndex_r3/Constant  const=1  equ=P=C  arith_type=Boolean  n_bits=8  bin_pt=0  opselect=C  inp2=PCIN>>17  opr=+  inp1=P  carry=CIN  iostate=0  explicit_period=on  period=1  dbl_ovrd=off
  Inverter{,1..3} (4 alike) : xbsIndex_r3/Inverter  latency=0  explicit_period=off  period=1  en=off  dbl_ovrd=off  show_param=off
      settings: xl_area=[0, 0, 0, 0, 0, 0, 0]
  Logical : xbsIndex_r3/Logical  logical_function=AND  inputs=2  precision=Full  arith_type=Unsigned  n_bits=8  bin_pt=2  align_bp=on  latency=0  explicit_period=off  period=1  en=off  dbl_ovrd=off  show_param=off
      settings: xl_area=[0, 0, 0, 0, 0, 0, 0]
  Logical1 : xbsIndex_r3/Logical  logical_function=AND  inputs=2  precision=Full  arith_type=Unsigned  n_bits=8  bin_pt=2  align_bp=on  latency=0  explicit_period=off  period=1  en=off  dbl_ovrd=off  show_param=off
      settings: xl_area=[0, 0, 0, 0, 0, 0, 0]
  Logical2 : xbsIndex_r3/Logical  logical_function=AND  inputs=2  precision=Full  arith_type=Unsigned  n_bits=8  bin_pt=2  align_bp=on  latency=0  explicit_period=off  period=1  en=off  dbl_ovrd=off  show_param=off
      settings: xl_area=[0, 0, 0, 0, 0, 0, 0]
  Register : xbsIndex_r3/Register  init=0  reg_only_valid=off  explicit_period=off  period=1  rst=on  en=on  out_en=off  dbl_ovrd=off  show_param=off
      settings: xl_area=[0, 0, 0, 0, 0, 0, 0]
  BRAM we : Outport
  wires:
  [valid] -> Inverter/1
  get_spec/1 -> Inverter2/1, Logical/1
  Inverter/1 -> Logical/2
  Constant1/1 -> Register/1
  Logical/1 -> Register/3
  Register/1 -> Inverter1/1
  Inverter1/1 -> Logical1/2
  Inverter2/1 -> Logical2/2
  Inverter3/1 -> Logical2/1
  Logical2/1 -> Register/2
  Logical1/1 -> BRAM we/1
  valid/1 -> [valid]
  [valid] -> Inverter3/1
  [valid] -> Logical1/1

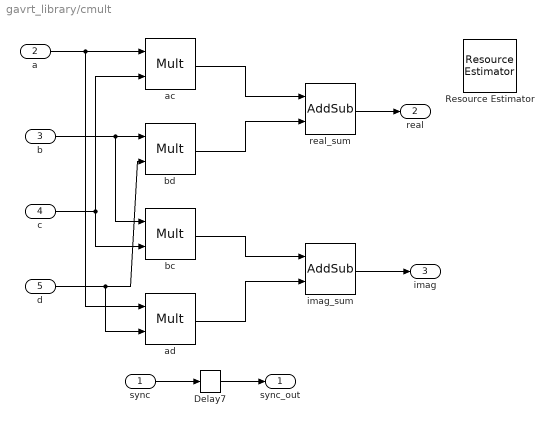
== system gavrt_library/cmult ==
  sync : Inport  Port=1  LatchInput=off
  a : Inport  Port=2  LatchInput=off
  b : Inport  Port=3  LatchInput=off
  c : Inport  Port=4  LatchInput=off
  d : Inport  Port=5  LatchInput=off
  Delay7 : xbsIndex_r3/Delay  latency=add_latency+mult_latency  reg_retiming=off  explicit_period=off  period=1  en=off  accept_only_valid=off  init_zero=on  dbl_ovrd=off  show_param=off
      settings: xl_area=[0, 0, 0, 0, 0, 0, 0]
  Resource Estimator : xbsIndex_r3/Resource Estimator  Tag=resEstTag  xl_estimator_area=[26 18 0 48 0 4 0]  xl_use_estimator_area=off  simulink_period=1  mrp_directory=W:\casper_work\scratch\adcxaui
      settings: AttributesFormatString=Resource\nEstimator
  ac : xbsIndex_r3/Mult  precision=Full  arith_type="Signed  (2's comp)"  n_bits=8  bin_pt=2  quantization=Truncate  overflow=Wrap  latency=mult_latency  explicit_period=off  period=1  en=off  dbl_ovrd=off  show_param=on  mult_type=Parallel  oversample=2  use_embedded=on  pipeline=on  use_rpm=on  placement_style=Rectangular Shape  gen_core=off
      settings: xl_area=[4 0 0 8 0 1 0]
  ad : xbsIndex_r3/Mult  precision=Full  arith_type="Signed  (2's comp)"  n_bits=8  bin_pt=2  quantization=Truncate  overflow=Wrap  latency=mult_latency  explicit_period=off  period=1  en=off  dbl_ovrd=off  show_param=on  mult_type=Parallel  oversample=2  use_embedded=on  pipeline=on  use_rpm=on  placement_style=Rectangular Shape  gen_core=off
      settings: xl_area=[4 0 0 8 0 1 0]
  bc : xbsIndex_r3/Mult  precision=Full  arith_type="Signed  (2's comp)"  n_bits=8  bin_pt=2  quantization=Truncate  overflow=Wrap  latency=mult_latency  explicit_period=off  period=1  en=off  dbl_ovrd=off  show_param=on  mult_type=Parallel  oversample=2  use_embedded=on  pipeline=on  use_rpm=on  placement_style=Rectangular Shape  gen_core=off
      settings: xl_area=[4 0 0 8 0 1 0]
  bd : xbsIndex_r3/Mult  precision=Full  arith_type="Signed  (2's comp)"  n_bits=8  bin_pt=2  quantization=Truncate  overflow=Wrap  latency=mult_latency  explicit_period=off  period=1  en=off  dbl_ovrd=off  show_param=on  mult_type=Parallel  oversample=2  use_embedded=on  pipeline=on  use_rpm=on  placement_style=Rectangular Shape  gen_core=off
      settings: xl_area=[4 0 0 8 0 1 0]
  imag_sum : xbsIndex_r3/AddSub  mode=Addition  precision=Full  arith_type=Unsigned  n_bits=8  bin_pt=2  quantization=Truncate  overflow=Wrap  latency=add_latency  explicit_period=off  period=1  use_carryin=off  use_carryout=off  en=off  dbl_ovrd=off  show_param=on  use_core=on  pipeline=on  use_rpm=on  gen_core=off
      settings: xl_area=[5 9 0 8 0 0 0]
  real_sum : xbsIndex_r3/AddSub  mode=Subtraction  precision=Full  arith_type=Unsigned  n_bits=8  bin_pt=2  quantization=Truncate  overflow=Wrap  latency=add_latency  explicit_period=off  period=1  use_carryin=off  use_carryout=off  en=off  dbl_ovrd=off  show_param=on  use_core=on  pipeline=on  use_rpm=on  gen_core=off
      settings: xl_area=[5 9 0 8 0 0 0]
  sync_out : Outport
  real : Outport  Port=2
  imag : Outport  Port=3
  wires:
  Delay7/1 -> sync_out/1
  sync/1 -> Delay7/1
  ac/1 -> real_sum/1
  bd/1 -> real_sum/2
  bc/1 -> imag_sum/1
  ad/1 -> imag_sum/2
  a/1 -> ad/1, ac/1
  c/1 -> bc/2, ac/2
  b/1 -> bc/1, bd/1
  d/1 -> ad/2, bd/2
  real_sum/1 -> real/1
  imag_sum/1 -> imag/1
